simulink model "exwaypointFollower"  (R2020a)
settings: Solver=VariableStepAuto  StartTime=0.0  StopTime=10.0  RelTol=1e-3
values from neighbouring files (symbols this model uses):
  robs = [3.0 1.0 1.1 0.5 1]    [CreateModel.m]    (also in MyCost.m = model.robs; SolnPlot.m = model.robs; pso.m = model.robs; test3.m = [1.5 1.0 0.8])
  xobs = [5.5 3.0 1.5 0.6 10]    [CreateModel.m]    (also in MyCost.m = model.xobs; SolnPlot.m = model.xobs; pso.m = model.xobs; test3.m = [1.5 4.0 1.2])
  xtri = model.xtri    [AreaofTriangle.m]    (also in CreateModel.m = [0 0 2]; MyCost.m; SolnPlot.m; pso.m)
  yobs = [7 4.0 1.2 3.5 7]    [CreateModel.m]    (also in MyCost.m = model.yobs; SolnPlot.m = model.yobs; pso.m = model.yobs; test3.m = [4.5 3.0 1.5])
  ytri = model.ytri    [AreaofTriangle.m]    (also in CreateModel.m = [7 5 6]; MyCost.m; SolnPlot.m; pso.m)
settings Model: Creator=Windows  LastModifiedBy=Windows

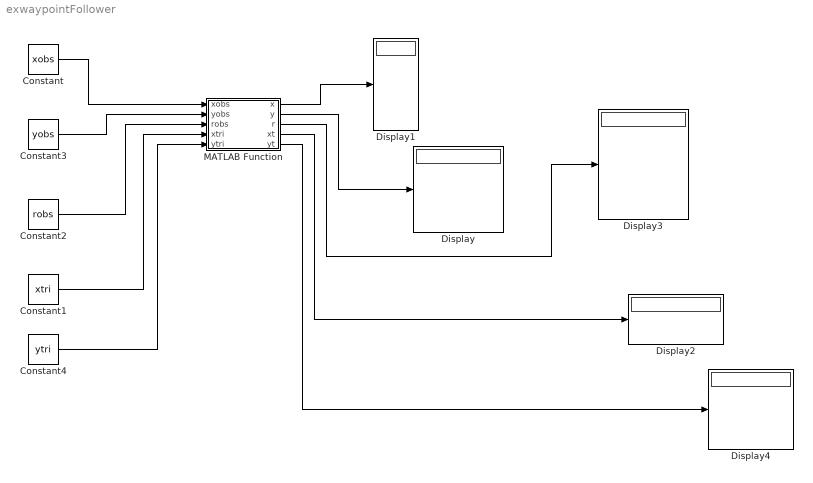
== system exwaypointFollower ==
  Constant : Constant  Value=xobs
  Constant1 : Constant  Value=xtri
  Constant2 : Constant  Value=robs
  Constant3 : Constant  Value=yobs
  Constant4 : Constant  Value=ytri
  Display{,1..4} (5 alike) : Display
  MATLAB Function : MATLAB Function  TreatAsAtomicUnit=on
  wires:
  Constant/1 -> MATLAB Function/1(xobs)
  Constant3/1 -> MATLAB Function/2(yobs)
  Constant2/1 -> MATLAB Function/3(robs)
  Constant1/1 -> MATLAB Function/4(xtri)
  Constant4/1 -> MATLAB Function/5(ytri)
  MATLAB Function/1(x) -> Display1/1
  MATLAB Function/2(y) -> Display/1
  MATLAB Function/3(r) -> Display3/1
  MATLAB Function/4(xt) -> Display2/1
  MATLAB Function/5(yt) -> Display4/1

== matlab function exwaypointFollower/MATLAB Function ==
  data: xobs input; x output; y output; yobs input; robs input; xtri input; ytri input; r output; xt output; yt output
function [x,y,r,xt,yt] = fcn(xobs,yobs,robs,xtri,ytri)

    x= xobs;
    y= yobs;
    r= robs;
    xt= xtri;
    yt= ytri;
    a=[1,1 ,1];
    T=[1 ,0,0;0,1,0;0,0,1];

theta=linspace(0,2*pi,100);
    for k=1:numel(x)
        plot(x(k)+r(k)*cos(theta),y(k)+r(k)*sin(theta),'ro');
        hold on;
    end
    
    for k=1:numel(xt)
        if(k==3)
             theta1=transpose(linspace(xt(k),xt(1),100));
              theta2=transpose(linspace(yt(k),yt(1),100));
              
        
        else
        theta1=transpose(linspace(xt(k),xt(k+1),100));
        theta2=transpose(linspace(yt(k),yt(k+1),100));
        end
    
        if(xt(k)>xt(k+1))
    plot(xt(k)+theta1,yt(k)+theta2,'bo');
    
       plot(xt(k),yt(k),'ro');
        end
       triplot(T,xt,yt);
    end
